simulink model "quadplane_controlA"  (R2023a)
settings: Solver=FixedStepAuto  StartTime=0.0  StopTime=10.0  FixedStep=0.001  RelTol=1e-3
undefined symbols (not defined in the file): Aircraft, framePeriod_s, frameRate_hz
libraries: simulink x12, slpidlib x1, fuzblock x1
(part 2 of 2)

== system quadplane_controlA/FixedWing OuterLoop Control/INDI Speed & Altitude Controller/LowPass Filter ==
  raw_val : Inport
  Constant : Constant  Value=Aircraft.Control.Forward.outer_indi_outputs_LP_filter_CTOFF  OutDataTypeStr=single
  LP Filter on Accel : Subsystem
      settings: PortSchema="{\"entries\":[{\"content\":{\"sides\":[{\"content\":{\"connectorIds\":[\"In1\"]},\"type\":\"ConnectorPlacement.EquallySpacedRectSide\",\"uuid\":\"20236834-aeb3-4c5b-bb2e-f84447e752b5\"},{\"content\":{\"connectorIds\":[\"Out1\"],\"side\":\"RIGHT\"},\"type\":\"ConnectorPlacement.EquallySpacedRectSide\",\"uuid\":\"d668f9a1-a3df-4207-8bf1-99fb838e59b2\"},{\"content\":{\"connectorIds\":[],\"side\":\"TOP\"},\"type\":\"ConnectorPlacement.EquallySpacedRectSide\",\"uuid\":\"66cceb06-f4bc-4278-b965-2427292e46df\"},{\"content\":{\"connectorIds\":[\"In2\"],\"side\":\"BOTTOM\"},\"type\":\"ConnectorPlacement.EquallySpacedRectSide\",\"uuid\":\"8fdaac6a-cb03-4bd4-87bb-7bafd10bc297\"}]},\"type\":\"ConnectorPlacement.EquallySpacedConnector\",\"uuid\":\"3dc29a9a-e794-478d-b7df-452e6c2d3f66\"}],\"packageUris\":[\"http://schema.mathworks.com/mf0/Connector/R2020b\"],\"version\":\"1.0\"}"
  filtered_val : Outport
  wires:
  raw_val/1 -> LP Filter on Accel/1(raw_val)
  Constant/1 -> LP Filter on Accel/2(freq_cut)
  LP Filter on Accel/1(filtered_val) -> filtered_val/1

== system quadplane_controlA/FixedWing OuterLoop Control/INDI Speed & Altitude Controller/LowPass Filter1 ==
  raw_val : Inport
  Constant : Constant  Value=Aircraft.Control.Hover.u_ref_LP_filter_CTOFF
  LP Filter on throttle outputs : Subsystem
      settings: PortSchema="{\"entries\":[{\"content\":{\"sides\":[{\"content\":{\"connectorIds\":[\"In1\"]},\"type\":\"ConnectorPlacement.EquallySpacedRectSide\",\"uuid\":\"20236834-aeb3-4c5b-bb2e-f84447e752b5\"},{\"content\":{\"connectorIds\":[\"Out1\"],\"side\":\"RIGHT\"},\"type\":\"ConnectorPlacement.EquallySpacedRectSide\",\"uuid\":\"d668f9a1-a3df-4207-8bf1-99fb838e59b2\"},{\"content\":{\"connectorIds\":[],\"side\":\"TOP\"},\"type\":\"ConnectorPlacement.EquallySpacedRectSide\",\"uuid\":\"66cceb06-f4bc-4278-b965-2427292e46df\"},{\"content\":{\"connectorIds\":[\"In2\"],\"side\":\"BOTTOM\"},\"type\":\"ConnectorPlacement.EquallySpacedRectSide\",\"uuid\":\"8fdaac6a-cb03-4bd4-87bb-7bafd10bc297\"}]},\"type\":\"ConnectorPlacement.EquallySpacedConnector\",\"uuid\":\"3dc29a9a-e794-478d-b7df-452e6c2d3f66\"}],\"packageUris\":[\"http://schema.mathworks.com/mf0/Connector/R2020b\"],\"version\":\"1.0\"}"
  filtered_val : Outport
  wires:
  raw_val/1 -> LP Filter on throttle outputs/1(raw_val)
  Constant/1 -> LP Filter on throttle outputs/2(freq_cut)
  LP Filter on throttle outputs/1(filtered_val) -> filtered_val/1

== system quadplane_controlA/Hover Inner Loop/INDI inner loop/LowPass Filter ==
  raw_val : Inport
  Constant : Constant  Value=Aircraft.Control.Hover.throttle_output_LP_filter_CTOFF
  LP Filter on throttle outputs : Subsystem
      settings: PortSchema="{\"entries\":[{\"content\":{\"sides\":[{\"content\":{\"connectorIds\":[\"In1\"]},\"type\":\"ConnectorPlacement.EquallySpacedRectSide\",\"uuid\":\"20236834-aeb3-4c5b-bb2e-f84447e752b5\"},{\"content\":{\"connectorIds\":[\"Out1\"],\"side\":\"RIGHT\"},\"type\":\"ConnectorPlacement.EquallySpacedRectSide\",\"uuid\":\"d668f9a1-a3df-4207-8bf1-99fb838e59b2\"},{\"content\":{\"connectorIds\":[],\"side\":\"TOP\"},\"type\":\"ConnectorPlacement.EquallySpacedRectSide\",\"uuid\":\"66cceb06-f4bc-4278-b965-2427292e46df\"},{\"content\":{\"connectorIds\":[\"In2\"],\"side\":\"BOTTOM\"},\"type\":\"ConnectorPlacement.EquallySpacedRectSide\",\"uuid\":\"8fdaac6a-cb03-4bd4-87bb-7bafd10bc297\"}]},\"type\":\"ConnectorPlacement.EquallySpacedConnector\",\"uuid\":\"3dc29a9a-e794-478d-b7df-452e6c2d3f66\"}],\"packageUris\":[\"http://schema.mathworks.com/mf0/Connector/R2020b\"],\"version\":\"1.0\"}"
  filtered_val : Outport
  wires:
  raw_val/1 -> LP Filter on throttle outputs/1(raw_val)
  Constant/1 -> LP Filter on throttle outputs/2(freq_cut)
  LP Filter on throttle outputs/1(filtered_val) -> filtered_val/1

== system quadplane_controlA/Hover Inner Loop/INDI inner loop/LowPass Filter1 ==
  raw_val : Inport
  Constant : Constant  Value=Aircraft.Control.Hover.inner_ref_LP_filter_CTOFF
  LP Filter on throttle outputs : Subsystem
      settings: PortSchema="{\"entries\":[{\"content\":{\"sides\":[{\"content\":{\"connectorIds\":[\"In1\"]},\"type\":\"ConnectorPlacement.EquallySpacedRectSide\",\"uuid\":\"20236834-aeb3-4c5b-bb2e-f84447e752b5\"},{\"content\":{\"connectorIds\":[\"Out1\"],\"side\":\"RIGHT\"},\"type\":\"ConnectorPlacement.EquallySpacedRectSide\",\"uuid\":\"d668f9a1-a3df-4207-8bf1-99fb838e59b2\"},{\"content\":{\"connectorIds\":[],\"side\":\"TOP\"},\"type\":\"ConnectorPlacement.EquallySpacedRectSide\",\"uuid\":\"66cceb06-f4bc-4278-b965-2427292e46df\"},{\"content\":{\"connectorIds\":[\"In2\"],\"side\":\"BOTTOM\"},\"type\":\"ConnectorPlacement.EquallySpacedRectSide\",\"uuid\":\"8fdaac6a-cb03-4bd4-87bb-7bafd10bc297\"}]},\"type\":\"ConnectorPlacement.EquallySpacedConnector\",\"uuid\":\"3dc29a9a-e794-478d-b7df-452e6c2d3f66\"}],\"packageUris\":[\"http://schema.mathworks.com/mf0/Connector/R2020b\"],\"version\":\"1.0\"}"
  filtered_val : Outport
  wires:
  raw_val/1 -> LP Filter on throttle outputs/1(raw_val)
  Constant/1 -> LP Filter on throttle outputs/2(freq_cut)
  LP Filter on throttle outputs/1(filtered_val) -> filtered_val/1

== system quadplane_controlA/Subsystem/Subsystem1/Subsystem ==
  advance_waypoint : Inport
  motors_enabled : Inport  Port=2
  mode : Inport  Port=3
  sbus : Inport  Port=4
  pwm : Inport  Port=5
  throttle_cmd_prcnt : Inport  Port=6
  flight_time_remaining_s : Inport  Port=7
  power_remaining_prcnt : Inport  Port=8
  aux : Inport  Port=9
  Bus Creator : BusCreator  Inputs=9  OutDataTypeStr=Bus: VmsData  NonVirtualBus=on
      settings: InheritFromInputs=off
  vmsdata : Outport
  wires:
  flight_time_remaining_s/1 -> Bus Creator/7  "flight_time_remaining_s"
  mode/1 -> Bus Creator/3  "mode"
  pwm/1 -> Bus Creator/5  "pwm"
  aux/1 -> Bus Creator/9  "aux"
  throttle_cmd_prcnt/1 -> Bus Creator/6  "throttle_cmd_prcnt"
  Bus Creator/1 -> vmsdata/1
  motors_enabled/1 -> Bus Creator/2  "motors_enabled"
  advance_waypoint/1 -> Bus Creator/1  "advance_waypoint"
  power_remaining_prcnt/1 -> Bus Creator/8  "power_remaining_prcnt"
  sbus/1 -> Bus Creator/4  "sbus"

== system quadplane_controlA/Enabled Subsystem/Speed Control/LowPass Filter1/LP Filter on throttle outputs ==
  raw_val : Inport
  freq_cut : Inport  Port=2
  Constant : Constant  Value=frameRate_hz  OutDataTypeStr=single
  MATLAB Function : MATLAB Function  TreatAsAtomicUnit=on
  Unit Delay : UnitDelay  SampleTime=-1  HasFrameUpgradeWarning=on
  filtered_val : Outport
  wires:
  freq_cut/1 -> MATLAB Function/3(freq_cut)
  MATLAB Function/1(filtered_val) -> Unit Delay/1, filtered_val/1
  Unit Delay/1 -> MATLAB Function/1(prev_val)
  raw_val/1 -> MATLAB Function/2(raw_val)
  Constant/1 -> MATLAB Function/4(samp_freq)

== system quadplane_controlA/Enabled Subsystem/Speed Control/LowPass Filter2/LP Filter on throttle outputs ==
  raw_val : Inport
  freq_cut : Inport  Port=2
  Constant : Constant  Value=frameRate_hz  OutDataTypeStr=single
  MATLAB Function : MATLAB Function  TreatAsAtomicUnit=on
  Unit Delay : UnitDelay  SampleTime=-1  HasFrameUpgradeWarning=on
  filtered_val : Outport
  wires:
  freq_cut/1 -> MATLAB Function/3(freq_cut)
  MATLAB Function/1(filtered_val) -> Unit Delay/1, filtered_val/1
  Unit Delay/1 -> MATLAB Function/1(prev_val)
  raw_val/1 -> MATLAB Function/2(raw_val)
  Constant/1 -> MATLAB Function/4(samp_freq)

== system quadplane_controlA/FixedWing InnerLoop Control/INDI Based Angular Rate Controller/LowPass Filter/LP Filter on throttle outputs ==
  raw_val : Inport
  freq_cut : Inport  Port=2
  Constant : Constant  Value=frameRate_hz  OutDataTypeStr=single
  MATLAB Function : MATLAB Function  TreatAsAtomicUnit=on
  Unit Delay : UnitDelay  SampleTime=-1  HasFrameUpgradeWarning=on
  filtered_val : Outport
  wires:
  freq_cut/1 -> MATLAB Function/3(freq_cut)
  MATLAB Function/1(filtered_val) -> Unit Delay/1, filtered_val/1
  Unit Delay/1 -> MATLAB Function/1(prev_val)
  raw_val/1 -> MATLAB Function/2(raw_val)
  Constant/1 -> MATLAB Function/4(samp_freq)

== system quadplane_controlA/FixedWing InnerLoop Control/INDI Based Angular Rate Controller/LowPass Filter1/LP Filter on throttle outputs ==
  raw_val : Inport
  freq_cut : Inport  Port=2
  Constant : Constant  Value=frameRate_hz  OutDataTypeStr=single
  MATLAB Function : MATLAB Function  TreatAsAtomicUnit=on
  Unit Delay : UnitDelay  SampleTime=-1  HasFrameUpgradeWarning=on
  filtered_val : Outport
  wires:
  freq_cut/1 -> MATLAB Function/3(freq_cut)
  MATLAB Function/1(filtered_val) -> Unit Delay/1, filtered_val/1
  Unit Delay/1 -> MATLAB Function/1(prev_val)
  raw_val/1 -> MATLAB Function/2(raw_val)
  Constant/1 -> MATLAB Function/4(samp_freq)

== system quadplane_controlA/FixedWing InnerLoop Control/NDI based Attitude Controller/SideSlip Controller/LowPass Filter ==
  raw_val : Inport
  Constant : Constant  Value=Aircraft.Control.sideslip_ctrl.accel_LP_filter_CTOFF
  LP Filter on Accel : Subsystem
      settings: PortSchema="{\"entries\":[{\"content\":{\"sides\":[{\"content\":{\"connectorIds\":[\"In1\"]},\"type\":\"ConnectorPlacement.EquallySpacedRectSide\",\"uuid\":\"20236834-aeb3-4c5b-bb2e-f84447e752b5\"},{\"content\":{\"connectorIds\":[\"Out1\"],\"side\":\"RIGHT\"},\"type\":\"ConnectorPlacement.EquallySpacedRectSide\",\"uuid\":\"d668f9a1-a3df-4207-8bf1-99fb838e59b2\"},{\"content\":{\"connectorIds\":[],\"side\":\"TOP\"},\"type\":\"ConnectorPlacement.EquallySpacedRectSide\",\"uuid\":\"66cceb06-f4bc-4278-b965-2427292e46df\"},{\"content\":{\"connectorIds\":[\"In2\"],\"side\":\"BOTTOM\"},\"type\":\"ConnectorPlacement.EquallySpacedRectSide\",\"uuid\":\"8fdaac6a-cb03-4bd4-87bb-7bafd10bc297\"}]},\"type\":\"ConnectorPlacement.EquallySpacedConnector\",\"uuid\":\"3dc29a9a-e794-478d-b7df-452e6c2d3f66\"}],\"packageUris\":[\"http://schema.mathworks.com/mf0/Connector/R2020b\"],\"version\":\"1.0\"}"
  filtered_val : Outport
  wires:
  raw_val/1 -> LP Filter on Accel/1(raw_val)
  Constant/1 -> LP Filter on Accel/2(freq_cut)
  LP Filter on Accel/1(filtered_val) -> filtered_val/1

== system quadplane_controlA/FixedWing OuterLoop Control/INDI Speed & Altitude Controller/LowPass Filter/LP Filter on Accel ==
  raw_val : Inport
  freq_cut : Inport  Port=2
  Constant : Constant  Value=frameRate_hz  OutDataTypeStr=single
  MATLAB Function : MATLAB Function  TreatAsAtomicUnit=on
  Unit Delay : UnitDelay  SampleTime=-1  HasFrameUpgradeWarning=on
  filtered_val : Outport
  wires:
  freq_cut/1 -> MATLAB Function/3(freq_cut)
  MATLAB Function/1(filtered_val) -> Unit Delay/1, filtered_val/1
  Unit Delay/1 -> MATLAB Function/1(prev_val)
  raw_val/1 -> MATLAB Function/2(raw_val)
  Constant/1 -> MATLAB Function/4(samp_freq)

== system quadplane_controlA/FixedWing OuterLoop Control/INDI Speed & Altitude Controller/LowPass Filter1/LP Filter on throttle outputs ==
  raw_val : Inport
  freq_cut : Inport  Port=2
  Constant : Constant  Value=frameRate_hz  OutDataTypeStr=single
  MATLAB Function : MATLAB Function  TreatAsAtomicUnit=on
  Unit Delay : UnitDelay  SampleTime=-1  HasFrameUpgradeWarning=on
  filtered_val : Outport
  wires:
  freq_cut/1 -> MATLAB Function/3(freq_cut)
  MATLAB Function/1(filtered_val) -> Unit Delay/1, filtered_val/1
  Unit Delay/1 -> MATLAB Function/1(prev_val)
  raw_val/1 -> MATLAB Function/2(raw_val)
  Constant/1 -> MATLAB Function/4(samp_freq)

== system quadplane_controlA/Hover Inner Loop/INDI inner loop/LowPass Filter/LP Filter on throttle outputs ==
  raw_val : Inport
  freq_cut : Inport  Port=2
  Constant : Constant  Value=frameRate_hz  OutDataTypeStr=single
  MATLAB Function : MATLAB Function  TreatAsAtomicUnit=on
  Unit Delay : UnitDelay  SampleTime=-1  HasFrameUpgradeWarning=on
  filtered_val : Outport
  wires:
  freq_cut/1 -> MATLAB Function/3(freq_cut)
  MATLAB Function/1(filtered_val) -> Unit Delay/1, filtered_val/1
  Unit Delay/1 -> MATLAB Function/1(prev_val)
  raw_val/1 -> MATLAB Function/2(raw_val)
  Constant/1 -> MATLAB Function/4(samp_freq)

== system quadplane_controlA/Hover Inner Loop/INDI inner loop/LowPass Filter1/LP Filter on throttle outputs ==
  raw_val : Inport
  freq_cut : Inport  Port=2
  Constant : Constant  Value=frameRate_hz  OutDataTypeStr=single
  MATLAB Function : MATLAB Function  TreatAsAtomicUnit=on
  Unit Delay : UnitDelay  SampleTime=-1  HasFrameUpgradeWarning=on
  filtered_val : Outport
  wires:
  freq_cut/1 -> MATLAB Function/3(freq_cut)
  MATLAB Function/1(filtered_val) -> Unit Delay/1, filtered_val/1
  Unit Delay/1 -> MATLAB Function/1(prev_val)
  raw_val/1 -> MATLAB Function/2(raw_val)
  Constant/1 -> MATLAB Function/4(samp_freq)

== system quadplane_controlA/FixedWing InnerLoop Control/NDI based Attitude Controller/SideSlip Controller/LowPass Filter/LP Filter on Accel ==
  raw_val : Inport
  freq_cut : Inport  Port=2
  Constant : Constant  Value=frameRate_hz  OutDataTypeStr=single
  MATLAB Function : MATLAB Function  TreatAsAtomicUnit=on
  Unit Delay : UnitDelay  SampleTime=-1  HasFrameUpgradeWarning=on
  filtered_val : Outport
  wires:
  freq_cut/1 -> MATLAB Function/3(freq_cut)
  MATLAB Function/1(filtered_val) -> Unit Delay/1, filtered_val/1
  Unit Delay/1 -> MATLAB Function/1(prev_val)
  raw_val/1 -> MATLAB Function/2(raw_val)
  Constant/1 -> MATLAB Function/4(samp_freq)

== matlab function quadplane_controlA/Hover Inner Loop/INDI inner loop/LowPass Filter/LP Filter on throttle outputs/MATLAB Function ==
  data: prev_val input single; raw_val input; filtered_val output; freq_cut input; samp_freq input
function filtered_val = IIR_filt( prev_val,raw_val, freq_cut, samp_freq)
    fc = freq_cut/samp_freq;
    b = 2 - cos(2 * pi * fc) - sqrt((2 - cos(2 * pi * fc))^2 - 1);
    a = 1 - b;
    filtered_val = a * raw_val + b * prev_val;

== matlab function quadplane_controlA/FixedWing InnerLoop Control/INDI Based Angular Rate Controller/Calculate incremental term from INDI equation ==
  data: dynamic_pressure input; Sref input; bref input; cref input; Cl_coefs input; Cm_coefs input; Cn_coefs input; B_mat output single; inertia_matrix_inv input single
function B_mat = incremental_control_term(dynamic_pressure, Sref, bref, cref, Cl_coefs, Cm_coefs, Cn_coefs, inertia_matrix_inv)

% Format of the coefficients array is:: 
% [base_val, alpha, beta, p, q, r, aileron_def, elevator_def, rudder_def]

% deflections are [ail, elev, rudder]

% CY, Cl, Cn are functions of (beta, p, q, r, aileron_def, rudder_def)

% g(x) = inv(I) * moment contributions due to surface deflections
% this function calculates partial derivative of g wrt u (Jacobian). 

% just the jacobian with the coefficents and deflections
jacobian_g_wrt_u = [Cl_coefs(7), 0, Cl_coefs(9);...
    0, Cm_coefs(8), 0; ...
    Cn_coefs(7), 0, Cn_coefs(9)];

% including the total moments 
B_mat = inertia_matrix_inv * Sref * dynamic_pressure .* ...
    [bref, cref, bref]' .* jacobian_g_wrt_u;

== matlab function quadplane_controlA/FixedWing InnerLoop Control/NDI based Attitude Controller/SideSlip Controller/LowPass Filter/LP Filter on Accel/MATLAB Function ==
  data: prev_val input single; raw_val input; filtered_val output; freq_cut input; samp_freq input
function filtered_val = IIR_filt( prev_val,raw_val, freq_cut, samp_freq)
    fc = freq_cut/samp_freq;
    b = 2 - cos(2 * pi * fc) - sqrt((2 - cos(2 * pi * fc))^2 - 1);
    a = 1 - b;
    filtered_val = a * raw_val + b * prev_val;

== matlab function quadplane_controlA/FixedWing OuterLoop Control/INDI Speed & Altitude Controller/MATLAB Function1 ==
  data: B0_mat input; x_ref_dot input; Kp_err_term input; del_u output; x_dot input
function del_u = incremental_output(B0_mat, x_ref_dot, Kp_err_term, x_dot)

% output equation of incremental INDI
del_u = B0_mat \ reshape((- x_dot + Kp_err_term + x_ref_dot), [2,1]);

== matlab function quadplane_controlA/FixedWing InnerLoop Control/INDI Based Angular Rate Controller/LowPass Filter/LP Filter on throttle outputs/MATLAB Function ==
  data: prev_val input single; raw_val input; filtered_val output; freq_cut input; samp_freq input
function filtered_val = IIR_filt( prev_val,raw_val, freq_cut, samp_freq)
    fc = freq_cut/samp_freq;
    b = 2 - cos(2 * pi * fc) - sqrt((2 - cos(2 * pi * fc))^2 - 1);
    a = 1 - b;
    filtered_val = a * raw_val + b * prev_val;

== matlab function quadplane_controlA/Enabled Subsystem/Speed Control/MATLAB Function ==
  data: roll_pitch input; B0_mat output; g input
function B0_mat = inversion_mat(roll_pitch, g)

roll = roll_pitch(1);
pitch = roll_pitch(2);

B0_mat = [0, -g*cos(pitch); g*cos(roll)*cos(pitch), -g*sin(roll)*sin(pitch)];

== matlab function quadplane_controlA/Enabled Subsystem/Speed Control/MATLAB Function1 ==
  data: B0_mat input; y_ref_rate input; del_u output; error_term input; x_rate input
function del_u = indi_eqn(B0_mat, y_ref_rate, error_term, x_rate)

del_u = B0_mat \ (-x_rate + error_term + y_ref_rate);

== matlab function quadplane_controlA/Enabled Subsystem/Altitude Control/MATLAB Function ==
  data: roll_pitch input; w_ref output; z_dot_nav_ref input
function w_ref = correct_att(roll_pitch, z_dot_nav_ref)

w_ref = z_dot_nav_ref / (cos(roll_pitch(1)) * cos(roll_pitch(2)));

== matlab function quadplane_controlA/Hover Inner Loop/INDI inner loop/LowPass Filter1/LP Filter on throttle outputs/MATLAB Function ==
  data: prev_val input single; raw_val input; filtered_val output; freq_cut input; samp_freq input
function filtered_val = IIR_filt( prev_val,raw_val, freq_cut, samp_freq)
    fc = freq_cut/samp_freq;
    b = 2 - cos(2 * pi * fc) - sqrt((2 - cos(2 * pi * fc))^2 - 1);
    a = 1 - b;
    filtered_val = a * raw_val + b * prev_val;

== matlab function quadplane_controlA/Subsystem/motor_PWM_denormalize/remap ==
  data: norm_in input; raw_out output; in_min input; in_max input; out_min input; out_max input
function raw_out = remap(norm_in,in_min,in_max,out_min,out_max)
raw_out = (norm_in - in_min) * (out_max - out_min)/(in_max-in_min) + out_min;

== matlab function quadplane_controlA/Enabled Subsystem/Speed Control/LowPass Filter1/LP Filter on throttle outputs/MATLAB Function ==
  data: prev_val input single; raw_val input; filtered_val output; freq_cut input; samp_freq input
function filtered_val = IIR_filt( prev_val,raw_val, freq_cut, samp_freq)
    fc = freq_cut/samp_freq;
    b = 2 - cos(2 * pi * fc) - sqrt((2 - cos(2 * pi * fc))^2 - 1);
    a = 1 - b;
    filtered_val = a * raw_val + b * prev_val;

== matlab function quadplane_controlA/Enabled Subsystem/Speed Control/LowPass Filter2/LP Filter on throttle outputs/MATLAB Function ==
  data: prev_val input single; raw_val input; filtered_val output; freq_cut input; samp_freq input
function filtered_val = IIR_filt( prev_val,raw_val, freq_cut, samp_freq)
    fc = freq_cut/samp_freq;
    b = 2 - cos(2 * pi * fc) - sqrt((2 - cos(2 * pi * fc))^2 - 1);
    a = 1 - b;
    filtered_val = a * raw_val + b * prev_val;

== matlab function quadplane_controlA/FixedWing OuterLoop Control/INDI Speed & Altitude Controller/LowPass Filter/LP Filter on Accel/MATLAB Function ==
  data: prev_val input single; raw_val input; filtered_val output; freq_cut input; samp_freq input
function filtered_val = IIR_filt( prev_val,raw_val, freq_cut, samp_freq)
    fc = freq_cut ./ samp_freq;
    b = 2 - cos(2 * pi .* fc) - sqrt((2 - cos(2 * pi .* fc)).^2 - 1);
    a = 1 - b;
    filtered_val = a .* raw_val + b .* prev_val;

== matlab function quadplane_controlA/Mode Selection ==
  data: airspeed_cmd input; mode_input input; enable_hover output; enable_forward output; mode output; sensors_active input; airspeed input; mode_shutoff_airspeeds input
function [enable_hover, enable_forward, mode] = mode_selector(airspeed_cmd, mode_input, sensors_active, airspeed, mode_shutoff_airspeeds)


if (sensors_active && mode_input==0)
    % Enable only Hover mode
    enable_hover = 1;
    enable_forward = 0;
    mode = 0;

elseif (sensors_active && mode_input==2)
    % Enable only forward flight mode
    enable_hover = 0;
    enable_forward = 1; 
    mode = 2; 

elseif (sensors_active && mode_input==1)
    
    if airspeed > mode_shutoff_airspeeds(2) && airspeed_cmd > mode_shutoff_airspeeds(2) + 1
        % disable hover motors after certain airspeed
        % operate purely as fixed-wing
        enable_hover = 0;
        enable_forward = 1;
        mode = 2;
    
    elseif airspeed < mode_shutoff_airspeeds(1) && airspeed_cmd < mode_shutoff_airspeeds(1) - 1
        % disable fixed wing stuff below certain airspeed
        % operate purely as quad
        enable_hover = 1;
        enable_forward = 0;
        mode = 0;
    
    else
        % actual transition phase
        enable_hover = 1;
        enable_forward = 1;
        mode = 1;

    end


elseif sensors_active && mode_input > 2

    error("Invalid mode selected ...")

else
    enable_hover = 0;
    enable_forward = 0;
    mode = 0;
  
end

== matlab function quadplane_controlA/Subsystem1/MATLAB Function ==
  data: alpha input; airspeed input; adj_hover_thr output; adj_forward_thr output; hover_throttle input; forward_throttle input; surface_def input; adj_surface_def output
function [adj_hover_thr, adj_forward_thr, adj_surface_def] = weight_mixer(alpha, airspeed, hover_throttle, forward_throttle, surface_def)

% % Sorta Deadband
% if (airspeed<5)
%     alpha = 0;
% elseif (airspeed>15)
%     alpha = 1;
% else
%     % do nothing
% end


adj_hover_thr = (1-alpha) .* hover_throttle;

% adj_forward_thr = alpha .* forward_throttle;
% adj_surface_def = alpha .* surface_def;

adj_forward_thr = forward_throttle;
adj_surface_def = surface_def;

== matlab function quadplane_controlA/Subsystem/deflections_PWM_denormalize/remap ==
  data: norm_in input; raw_out output; in_min input; in_max input; out_min input; out_max input
function raw_out = remap(norm_in,in_min,in_max,out_min,out_max)
raw_out = (norm_in - in_min) * (out_max - out_min)/(in_max-in_min) + out_min;

== matlab function quadplane_controlA/FixedWing OuterLoop Control/INDI Speed & Altitude Controller/LowPass Filter1/LP Filter on throttle outputs/MATLAB Function ==
  data: prev_val input single; raw_val input; filtered_val output; freq_cut input; samp_freq input
function filtered_val = IIR_filt( prev_val,raw_val, freq_cut, samp_freq)
    fc = freq_cut/samp_freq;
    b = 2 - cos(2 * pi * fc) - sqrt((2 - cos(2 * pi * fc))^2 - 1);
    a = 1 - b;
    filtered_val = a * raw_val + b * prev_val;

== matlab function quadplane_controlA/FixedWing InnerLoop Control/INDI Based Angular Rate Controller/LowPass Filter1/LP Filter on throttle outputs/MATLAB Function ==
  data: prev_val input single; raw_val input; filtered_val output; freq_cut input; samp_freq input
function filtered_val = IIR_filt( prev_val,raw_val, freq_cut, samp_freq)
    fc = freq_cut/samp_freq;
    b = 2 - cos(2 * pi * fc) - sqrt((2 - cos(2 * pi * fc))^2 - 1);
    a = 1 - b;
    filtered_val = a * raw_val + b * prev_val;

== matlab function quadplane_controlA/FixedWing InnerLoop Control/NDI based Attitude Controller/NDI for Attitude Control ==
  data: yaw_rate_ref input; sum_term input; pqr_cmd output; roll_pitch input
function pqr_cmd = inversion_func(yaw_rate_ref, sum_term, roll_pitch)

roll = roll_pitch(1);
pitch = roll_pitch(2);

N_att_rates_to_pqr = [1, 0, -sin(pitch); ...
    0, cos(roll), sin(roll)*cos(pitch); ...
    0, -sin(roll), cos(roll)*cos(pitch)];

pqr_cmd = N_att_rates_to_pqr * [sum_term; yaw_rate_ref];

== matlab function quadplane_controlA/FixedWing InnerLoop Control/INDI Based Angular Rate Controller/Calculate incremented input from INDI equation ==
  data: B_mat input; pqr_ref_dot input; del_u output; K_out input; pqr_dot input; yaw_damper input
function del_u = indi_input_calc(B_mat, pqr_ref_dot, K_out, pqr_dot, yaw_damper)

% INDI controller's change in output term
del_u = B_mat \ reshape((-pqr_dot + K_out + pqr_ref_dot), [3,1]);

% damping rudder output using the r-rate
del_u(3) = del_u(3) - yaw_damper * pqr_dot(3);

== matlab function quadplane_controlA/FixedWing InnerLoop Control/NDI based Attitude Controller/SideSlip Controller/Yaw Rate Cmd Coming from roll ==
  settings: updateMethod=DISCRETE  sampleTime=0.01
  data: accel_z input; yaw_rate_cmd output single; roll_angle input; airspeed input; flight_path input
function yaw_rate_cmd = yaw_rate_cmd_from_roll(accel_z, roll_angle, airspeed, flight_path)

yaw_rate_cmd = -accel_z * sin(roll_angle) / (airspeed * cos(flight_path));

== matlab function quadplane_controlA/Hover Inner Loop/INDI inner loop/MATLAB Function ==
  data: B0_mat input; motor_cmds output; x_ref_rate input; Kp_term input; x_rate input
function motor_cmds = indi_inner_control(B0_mat, x_ref_rate, Kp_term, x_rate)

% INDI output change equation
motor_cmds = B0_mat \ (-x_rate + Kp_term + x_ref_rate);

== matlab function quadplane_controlA/Hover Inner Loop/INDI inner loop/MATLAB Function1 ==
  data: mass input; cg_pos input; thrust_coefs input; B0_mat output; torque_coefs input; motor_pos input; new_inertia_inv input; motor_cmds input
function B0_mat = inversion_matrix(mass, cg_pos, thrust_coefs, torque_coefs, motor_pos, new_inertia_inv, motor_cmds)
% Included all moments modelled for hover flight

% Assumed thrust coefficient and torque coefficients are 2nd order. 
moment_arm = motor_pos - cg_pos';

% 2*a1*omega_i + a2
dummy_term = 2 * thrust_coefs(1) .* motor_cmds' + thrust_coefs(2);

% dummy term with respective y position of motor
row_1_term = - moment_arm(1:4, 2)' .* dummy_term;

% dummy term with respective x position of motor
row_2_term = moment_arm(1:4, 1)' .* dummy_term;

% 2*b1*omega_i + b2
row_3_term = [-1,-1,1,1] .* (2 * torque_coefs(1) .* motor_cmds' + torque_coefs(2));

% (-1/m)(2a1*omega_i+a2)
row_4_term = (-1/mass) * (dummy_term);

% inversion matrix for INDI
B0_mat = new_inertia_inv * [row_1_term; row_2_term; row_3_term; row_4_term];

== matlab function quadplane_controlA/MATLAB Function ==
  data: ned_vector input; rpy_euler input; body_vector output
function body_vector = ned2body(ned_vector, rpy_euler)

roll = rpy_euler(1);
pitch = rpy_euler(2);
yaw = rpy_euler(3);

% Rotation matrix from NED to Body frame
C_ned2body = [cos(pitch)*cos(yaw), cos(pitch)*sin(yaw), -sin(pitch); ...
    sin(roll)*sin(pitch)*cos(yaw)-cos(roll)*sin(yaw), ...
    sin(roll)*sin(pitch)*sin(yaw)+cos(roll)*cos(yaw), sin(roll)*cos(pitch);...
    cos(roll)*sin(pitch)*cos(yaw)+sin(roll)*sin(yaw), ...
    cos(roll)*sin(pitch)*sin(yaw)-sin(roll)*cos(yaw), cos(roll)*cos(pitch)];

body_vector = C_ned2body * ned_vector;

== matlab function quadplane_controlA/FixedWing OuterLoop Control/INDI Speed & Altitude Controller/Compute Inversion Matrix ==
  data: throttle_cmd input; pitch_cmd input single; diam input; B0_mat output single; mass input single; density input single; Sref input single; CD_alpha input single; CL_alpha input single; x input single
function B0_mat = inversion_term(throttle_cmd, pitch_cmd, diam, mass, density, Sref, CD_alpha, CL_alpha, x)

airspeed = x(1);
flight_path = x(2);

% Rough generalizations to make the inversion eqn simpler
RPM = 4000 * (2*pi/60);
R = (diam/2) * 0.0254;

% dg/du term from the Taylor series expansion of the state derivative
B0_mat = [(1/(2*mass)) * density*(RPM^2)*pi*(R^4)*cos(pitch_cmd-flight_path), ...
    (-density/(2*mass)) * ( (airspeed^2)*Sref*CD_alpha + (RPM^2)*pi*(R^4)*throttle_cmd*sin(pitch_cmd-flight_path) ); ...
    (1/(2*airspeed)) * (density*(RPM^2)*pi*(R^4)*sin(pitch_cmd-flight_path)), ...
    (density/2) * (airspeed*Sref*CL_alpha + (1/airspeed)*(RPM^2)*pi*(R^4)*throttle_cmd*cos(pitch_cmd-flight_path) ) ];
